simulink library "ox_lib"  (Simulink 7.5)
settings: Solver=ode45  SolverMode=SingleTasking  StartTime=0.0  StopTime=10.0  RelTol=1e-3
PostLoadFcn:
  | % Stub definitions for mask variables
  | delay_depth=16;
  | n_bits=8;
  | bin_pt=7;
libraries: xbsIndex_r4 x493, casper_library x127, casper_library_misc x2, xps_library x2, casper_library_delays x1
(part 1 of 5)
settings Model: Creator=mwagner  LastModifiedBy=jack

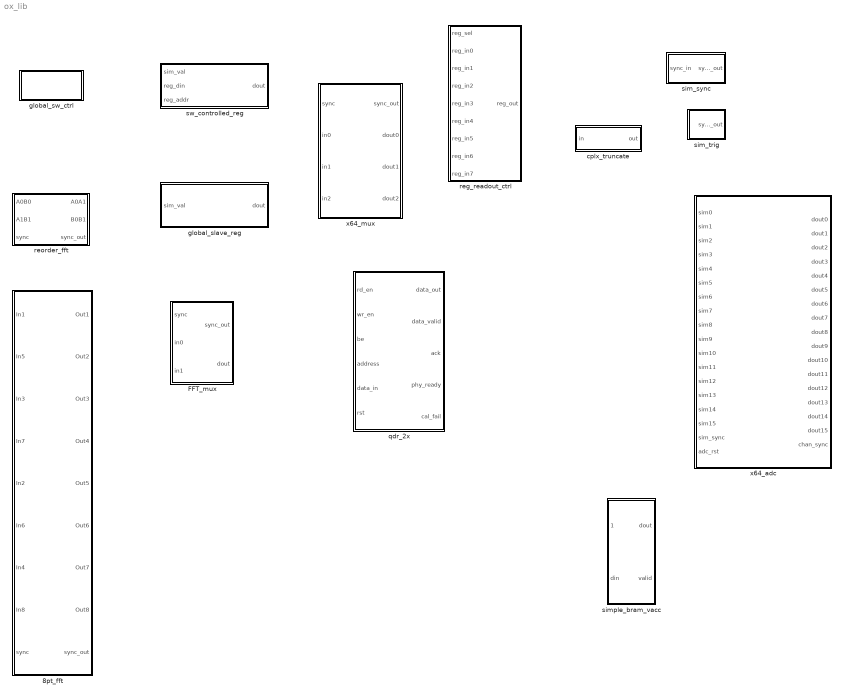
== system ox_lib ==
  8pt_fft : Subsystem
      mask Type: 8pt_fft
      mask Description:
      | Input 8 values and get 8 fourier components!
      | 
      | Simples!
      | 
      | [Latency 24]
  FFT_mux : Subsystem  mask{fft_len=9, fft_inputs=2, bit_width=18, bram_lat=2}
      mask prompts: fft_len "FFT length (2^?)"; fft_inputs "Number of FFT inputs (2^?) -- doesn't yet work for values other than 2"; bit_width "Bit width of samples"; bram_lat "bram latency"
  cplx_truncate : Subsystem  mask{in_bits=19, out_bits=16}
      mask prompts: in_bits "Input bitwidth"; out_bits "Output bitwidth"
  global_slave_reg : Subsystem  mask{reg_name=My Register, data_width=32, latency=0, auto=off, enable_bit=0}
      mask prompts: reg_name "Register Name"; data_width "Data width (bits): 1-32"; latency "Pipelined delay (0 for none)"; auto "Use automatic addressing? (not yet implemented)"; enable_bit "Address Number: 0-31"
      mask init:
      | pipeline_init([gcb '/pipeline1'], 'latency', latency);
      | pipeline_init([gcb '/pipeline2'], 'latency', latency);
      | 
      | fmtstr = sprintf('Name: %s, Number :%d, Latency:%d', reg_name, enable_bit, latency);
      | 
      | set_param(gcb, 'AttributesFormatString', fmtstr);
      settings: AttributesFormatString=Name: My Register, Number :0, Latency:10
  global_sw_ctrl : Subsystem
      settings: PermitHierarchicalResolution=None
      mask Type: global_sw_reg
      mask Description: The beginnings of a lightweight control system for designs with many software registers.
  qdr_2x : Subsystem  Tag=xps:qdr_2x  mask(qdr_2x){which_qdr=qdr0, qdr_awidth=12, use_sniffer=off}
      mask prompts: which_qdr "QDR Chip"; qdr_awidth "Simulation QDR address width"; use_sniffer "Include CPU Interface"
      mask help: Interface to the QDR II SRAM device on ROACH, with 2x multiplexing
      mask init:
      | qdr_2x_mask(gcb);
      mask StyleString: popup(qdr0|qdr1),edit,checkbox
  reg_readout_ctrl : Subsystem  mask{n_registers=8, mux_latency=2}
      mask prompts: n_registers "Number of register inputs"; mux_latency "mux latency"
      mask init:
      | reg_readout_ctrl_init(gcb, ...
      |     'n_registers', n_registers, ...
      |     'mux_latency', mux_latency);
      settings: AttributesFormatString=|
      | n_inputs=8
      | latency=2
  reorder_fft : Subsystem  mask{N=256}
      mask prompts: N "window size"
  sim_sync : Subsystem  mask{delay=1}
      mask prompts: delay "time of pulse (clocks from simulation start)"
  sim_trig : Subsystem  mask{delay=1}
      mask prompts: delay "time of pulse (clocks from simulation start)"
  simple_bram_vacc : Subsystem  mask(simple_bram_vacc){vec_len=8, arith_type=Signed, n_bits=32, bin_pt=0, acc_len=4}
      mask prompts: vec_len "Vector length:"; arith_type "Output type:"; n_bits "Bit width (output):"; bin_pt "Binary point (output):"; acc_len "Accumulation length?"
      mask help:
      | This simple vector accumulator is based on a shift register. It outputs its accumulated vector as soon as it is calculated.
      |
      | (I.e, it does not require a further new acc pulse, and therefore won't break if there are periods of invalid data)
      mask init:
      | simple_bram_vacc_init(gcb, ...
      |     'vec_len', vec_len, ...
      |     'arith_type', arith_type, ...
      |     'n_bits', n_bits, ...
      |     'bin_pt', bin_pt);
      | 
      | fmtstr = sprintf('Acc len: %d', acc_len);
      | set_param(gcb, 'AttributesFormatString', fmtstr);
      settings: AttributesFormatString=Acc len: 4
      mask StyleString: edit,popup(Signed|Unsigned),edit,edit,edit
  sw_controlled_reg : Subsystem  mask{reg_name=My Register, enable_bit=0, data_width=32}
      mask prompts: reg_name "Register Name"; enable_bit "Address Number: 0-31"; data_width "Data width (bits): 1-32"
      mask init:
      | fmtstr = sprintf('Name: %s\nNumber :%d', reg_name, enable_bit);
      | 
      | set_param(gcb, 'AttributesFormatString', fmtstr);
      settings: AttributesFormatString=|
      | Name: My Register
      | Number :0
  x64_adc : Subsystem  Tag=xps:x64_adc  mask(x64_adc){adc_clk_rate=64, spi=off, ctrl_gpio=GPIO_A}
      mask prompts: adc_clk_rate "ADC clock rate (MHz)"; spi "Include SPI interface?"; ctrl_gpio "GPIO bank to use for control signals?"
      mask help: The ADC block converts analog inputs to digital outputs. Every clock cycle, the inputs are sampled and digitized to 8 bit binary point numbers in the range of [-1, 1) and are then output by the adc.
      mask init:
      | x64_adc_mask(gcb);
      mask Help: eval('xlWeb([getenv(''MLIB_ROOT''), ''\doc\html\sys_adc\sys_adc.html''])')
      mask StyleString: edit,checkbox,popup(GPIO_A|GPIO_B)
  x64_mux : Subsystem  mask{fft_len=2, bram_lat=2}
      mask prompts: fft_len "FFT length (2^?)"; bram_lat "bram latency"

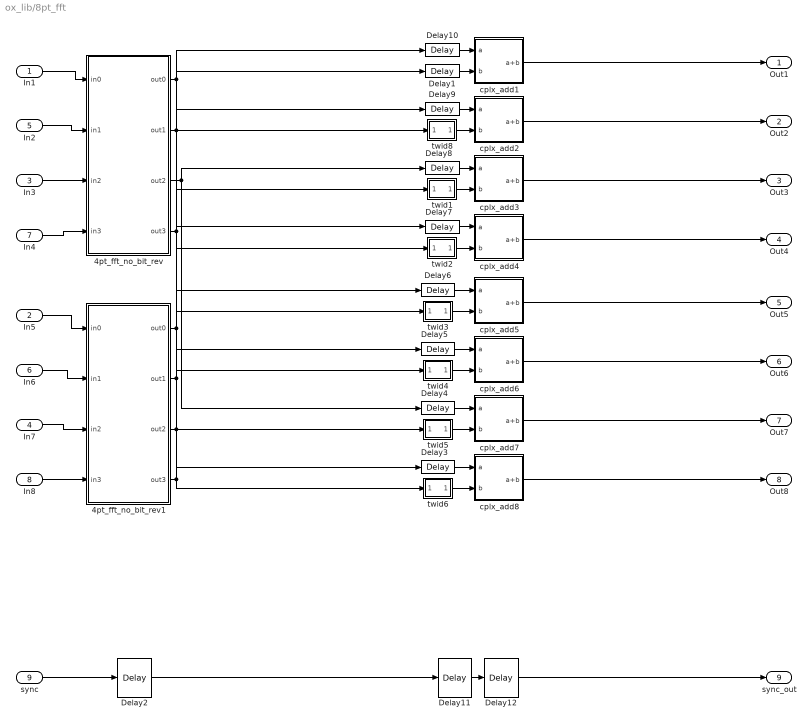
== system ox_lib/8pt_fft ==
  In1 : Inport  OutDataType=sfix(16)  OutScaling=2^0
  In5 : Inport  Port=2  OutDataType=sfix(16)  OutScaling=2^0
  In3 : Inport  Port=3  OutDataType=sfix(16)  OutScaling=2^0
  In7 : Inport  Port=4  OutDataType=sfix(16)  OutScaling=2^0
  In2 : Inport  Port=5  OutDataType=sfix(16)  OutScaling=2^0
  In6 : Inport  Port=6  OutDataType=sfix(16)  OutScaling=2^0
  In4 : Inport  Port=7  OutDataType=sfix(16)  OutScaling=2^0
  In8 : Inport  Port=8  OutDataType=sfix(16)  OutScaling=2^0
  sync : Inport  Port=9  OutDataType=sfix(16)  OutScaling=2^0
  4pt_fft_no_bit_rev : Subsystem
  4pt_fft_no_bit_rev1 : Subsystem
  Delay{1,3..11} (10 alike) : xbsIndex_r4/Delay  en=off  latency=8  dbl_ovrd=off  reg_retiming=off  block_type=delay
      settings: block_version=11.4
  Delay12 : xbsIndex_r4/Delay  en=off  latency=4  dbl_ovrd=off  reg_retiming=off  block_type=delay
      settings: block_version=11.4
  Delay2 : xbsIndex_r4/Delay  en=off  latency=12  dbl_ovrd=off  reg_retiming=off  block_type=delay
      settings: block_version=11.4
  cplx_add1 : Subsystem  AncestorBlock=casper_library/Misc/complex_addsub  mask(cplx_add){BitWidth=8, add_latency=2}
      mask prompts: BitWidth "Bit Wdith"; add_latency "Add Latency"
  cplx_add2 : Subsystem  AncestorBlock=casper_library/Misc/complex_addsub  mask(cplx_add){BitWidth=8, add_latency=2}
      mask prompts: BitWidth "Bit Wdith"; add_latency "Add Latency"
  cplx_add3 : Subsystem  AncestorBlock=casper_library/Misc/complex_addsub  mask(cplx_add){BitWidth=8, add_latency=2}
      mask prompts: BitWidth "Bit Wdith"; add_latency "Add Latency"
  cplx_add4 : Subsystem  AncestorBlock=casper_library/Misc/complex_addsub  mask(cplx_add){BitWidth=8, add_latency=2}
      mask prompts: BitWidth "Bit Wdith"; add_latency "Add Latency"
  cplx_add5 : Subsystem  AncestorBlock=casper_library/Misc/complex_addsub  mask(cplx_add){BitWidth=8, add_latency=2}
      mask prompts: BitWidth "Bit Wdith"; add_latency "Add Latency"
  cplx_add6 : Subsystem  AncestorBlock=casper_library/Misc/complex_addsub  mask(cplx_add){BitWidth=8, add_latency=2}
      mask prompts: BitWidth "Bit Wdith"; add_latency "Add Latency"
  cplx_add7 : Subsystem  AncestorBlock=casper_library/Misc/complex_addsub  mask(cplx_add){BitWidth=8, add_latency=2}
      mask prompts: BitWidth "Bit Wdith"; add_latency "Add Latency"
  cplx_add8 : Subsystem  AncestorBlock=casper_library/Misc/complex_addsub  mask(cplx_add){BitWidth=8, add_latency=2}
      mask prompts: BitWidth "Bit Wdith"; add_latency "Add Latency"
  twid1 : Subsystem  mask{phase=-2*pi/4}
      mask init:
      | fmtstr = sprintf('twiddle_phase: %d', phase);
      | set_param(gcb, 'AttributesFormatString', fmtstr);
      settings: AttributesFormatString=twiddle_phase: -1.570796e+00
  twid2 : Subsystem  mask{phase=-3*pi/4}
      mask init:
      | fmtstr = sprintf('twiddle_phase: %d', phase);
      | set_param(gcb, 'AttributesFormatString', fmtstr);
      settings: AttributesFormatString=twiddle_phase: -2.356194e+00
  twid3 : Subsystem  mask{phase=-4*pi/4}
      mask init:
      | fmtstr = sprintf('twiddle_phase: %d', phase);
      | set_param(gcb, 'AttributesFormatString', fmtstr);
      settings: AttributesFormatString=twiddle_phase: -3.141593e+00
  twid4 : Subsystem  mask{phase=-5*pi/4}
      mask init:
      | fmtstr = sprintf('twiddle_phase: %d', phase);
      | set_param(gcb, 'AttributesFormatString', fmtstr);
      settings: AttributesFormatString=twiddle_phase: -3.926991e+00
  twid5 : Subsystem  mask{phase=-6*pi/4}
      mask init:
      | fmtstr = sprintf('twiddle_phase: %d', phase);
      | set_param(gcb, 'AttributesFormatString', fmtstr);
      settings: AttributesFormatString=twiddle_phase: -4.712389e+00
  twid6 : Subsystem  mask{phase=-7*pi/4}
      mask init:
      | fmtstr = sprintf('twiddle_phase: %d', phase);
      | set_param(gcb, 'AttributesFormatString', fmtstr);
      settings: AttributesFormatString=twiddle_phase: -5.497787e+00
  twid8 : Subsystem  mask{phase=-pi/4}
      mask init:
      | fmtstr = sprintf('twiddle_phase: %d', phase);
      | set_param(gcb, 'AttributesFormatString', fmtstr);
      settings: AttributesFormatString=twiddle_phase: -7.853982e-01
  Out1 : Outport  OutDataType=sfix(16)  OutScaling=2^0
  Out2 : Outport  Port=2  OutDataType=sfix(16)  OutScaling=2^0
  Out3 : Outport  Port=3  OutDataType=sfix(16)  OutScaling=2^0
  Out4 : Outport  Port=4  OutDataType=sfix(16)  OutScaling=2^0
  Out5 : Outport  Port=5  OutDataType=sfix(16)  OutScaling=2^0
  Out6 : Outport  Port=6  OutDataType=sfix(16)  OutScaling=2^0
  Out7 : Outport  Port=7  OutDataType=sfix(16)  OutScaling=2^0
  Out8 : Outport  Port=8  OutDataType=sfix(16)  OutScaling=2^0
  sync_out : Outport  Port=9  OutDataType=sfix(16)  OutScaling=2^0
  wires:
  Delay10/1 -> cplx_add1/1(a)
  Delay9/1 -> cplx_add2/1(a)
  Delay8/1 -> cplx_add3/1(a)
  Delay7/1 -> cplx_add4/1(a)
  Delay6/1 -> cplx_add5/1(a)
  Delay5/1 -> cplx_add6/1(a)
  Delay4/1 -> cplx_add7/1(a)
  Delay3/1 -> cplx_add8/1(a)
  cplx_add8/1(a+b) -> Out8/1
  cplx_add7/1(a+b) -> Out7/1
  cplx_add6/1(a+b) -> Out6/1
  cplx_add5/1(a+b) -> Out5/1
  cplx_add4/1(a+b) -> Out4/1
  cplx_add3/1(a+b) -> Out3/1
  cplx_add2/1(a+b) -> Out2/1
  cplx_add1/1(a+b) -> Out1/1
  twid6/1(Out1) -> cplx_add8/2(b)
  twid5/1(Out1) -> cplx_add7/2(b)
  twid4/1(Out1) -> cplx_add6/2(b)
  twid3/1(Out1) -> cplx_add5/2(b)
  twid2/1(Out1) -> cplx_add4/2(b)
  twid1/1(Out1) -> cplx_add3/2(b)
  twid8/1(Out1) -> cplx_add2/2(b)
  Delay1/1 -> cplx_add1/2(b)
  sync/1 -> Delay2/1
  Delay2/1 -> Delay11/1
  Delay11/1 -> Delay12/1
  Delay12/1 -> sync_out/1
  In1/1 -> 4pt_fft_no_bit_rev/1(in0)
  In5/1 -> 4pt_fft_no_bit_rev1/1(in0)
  In6/1 -> 4pt_fft_no_bit_rev1/2(in1)
  In7/1 -> 4pt_fft_no_bit_rev1/3(in2)
  In8/1 -> 4pt_fft_no_bit_rev1/4(in3)
  4pt_fft_no_bit_rev/1(out0) -> Delay10/1, Delay6/1
  4pt_fft_no_bit_rev/2(out1) -> Delay9/1, Delay5/1
  4pt_fft_no_bit_rev/3(out2) -> Delay8/1, Delay4/1
  4pt_fft_no_bit_rev/4(out3) -> Delay7/1, Delay3/1
  4pt_fft_no_bit_rev1/1(out0) -> twid3/1(In1), Delay1/1
  4pt_fft_no_bit_rev1/2(out1) -> twid4/1(In1), twid8/1(In1)
  4pt_fft_no_bit_rev1/3(out2) -> twid5/1(In1), twid1/1(In1)
  4pt_fft_no_bit_rev1/4(out3) -> twid6/1(In1), twid2/1(In1)
  In2/1 -> 4pt_fft_no_bit_rev/2(in1)
  In3/1 -> 4pt_fft_no_bit_rev/3(in2)
  In4/1 -> 4pt_fft_no_bit_rev/4(in3)

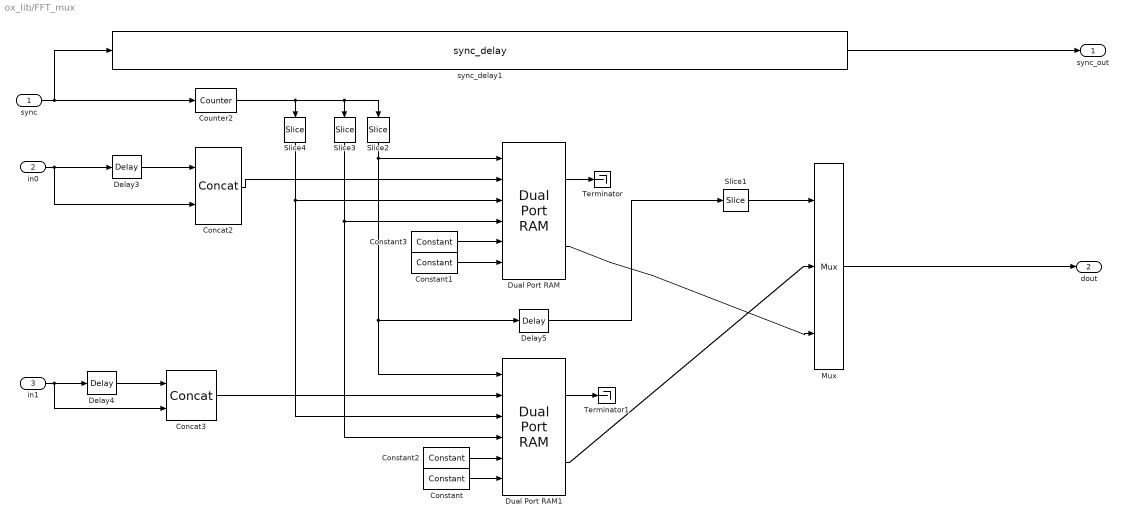
== system ox_lib/FFT_mux ==
  sync : Inport  OutDataType=fixdt(1, 16)  OutScaling=2^0
  in0 : Inport  Port=2  OutDataType=fixdt(1, 16)  OutScaling=2^0
  in1 : Inport  Port=3  OutDataType=fixdt(1, 16)  OutScaling=2^0
  Concat2 : xbsIndex_r4/Concat  num_inputs=2  dbl_ovrd=off  block_type=concat
  Concat3 : xbsIndex_r4/Concat  num_inputs=2  dbl_ovrd=off  block_type=concat
  Constant : xbsIndex_r4/Constant  arith_type=Boolean  const=0  n_bits=16  bin_pt=14  explicit_period=off  period=1  equ=P=C  opselect=C  inp2=PCIN>>17  opr=+  inp1=P  carry=CIN  dbl_ovrd=off  block_type=constant
      settings: block_version=11.4
  Constant1 : xbsIndex_r4/Constant  arith_type=Boolean  const=0  n_bits=16  bin_pt=14  explicit_period=off  period=1  equ=P=C  opselect=C  inp2=PCIN>>17  opr=+  inp1=P  carry=CIN  dbl_ovrd=off  block_type=constant
      settings: block_version=11.4
  Constant2 : xbsIndex_r4/Constant  arith_type=Unsigned  const=0  n_bits=(2^fft_inputs)*bit_width  bin_pt=0  explicit_period=on  period=1  equ=P=C  opselect=C  inp2=PCIN>>17  opr=+  inp1=P  carry=CIN  dbl_ovrd=off  block_type=constant
      settings: block_version=11.4
  Constant3 : xbsIndex_r4/Constant  arith_type=Unsigned  const=0  n_bits=(2^fft_inputs)*bit_width  bin_pt=0  explicit_period=on  period=1  equ=P=C  opselect=C  inp2=PCIN>>17  opr=+  inp1=P  carry=CIN  dbl_ovrd=off  block_type=constant
      settings: block_version=11.4
  Counter2 : xbsIndex_r4/Counter  cnt_type=Free Running  cnt_to=Inf  operation=Up  start_count=0  cnt_by_val=1  arith_type=Unsigned  n_bits=fft_len-fft_inputs+1  bin_pt=0  load_pin=off  rst=on  en=off  explicit_period=on  period=1  dbl_ovrd=off  use_behavioral_HDL=off  implementation=Fabric  block_type=counter
      settings: block_version=11.4
  Delay3 : xbsIndex_r4/Delay  en=off  latency=1  dbl_ovrd=off  reg_retiming=off  block_type=delay
      settings: block_version=11.4
  Delay4 : xbsIndex_r4/Delay  en=off  latency=1  dbl_ovrd=off  reg_retiming=off  block_type=delay
      settings: block_version=11.4
  Delay5 : xbsIndex_r4/Delay  en=off  latency=bram_lat  dbl_ovrd=off  reg_retiming=off  block_type=delay
      settings: block_version=11.4
  Dual Port RAM : xbsIndex_r4/Dual Port RAM  depth=2^(fft_len-fft_inputs)  initVector=0  distributed_mem=Block RAM  init_a=0  init_b=0  rst_a=off  rst_b=off  en_a=off  en_b=off  latency=bram_lat  write_mode_A=Read Before Write  write_mode_B=Read Before Write  dbl_ovrd=off  optimize=Area  use_rpm=on  block_type=dpram
      settings: block_version=11.4
  Dual Port RAM1 : xbsIndex_r4/Dual Port RAM  depth=2^(fft_len-fft_inputs)  initVector=0  distributed_mem=Block RAM  init_a=0  init_b=0  rst_a=off  rst_b=off  en_a=off  en_b=off  latency=bram_lat  write_mode_A=Read Before Write  write_mode_B=Read Before Write  dbl_ovrd=off  optimize=Area  use_rpm=on  block_type=dpram
      settings: block_version=11.4
  Mux : xbsIndex_r4/Mux  inputs=2  en=off  latency=1  precision=Full  arith_type=Unsigned  n_bits=16  bin_pt=14  quantization=Truncate  overflow=Wrap  dbl_ovrd=off  block_type=mux
      settings: block_version=11.4
  Slice1 : xbsIndex_r4/Slice  nbits=1  boolean_output=off  mode=Upper Bit Location + Width  bit1=0  base1=MSB of Input  bit0=0  base0=LSB of Input  dbl_ovrd=off  block_type=slice
  Slice2 : xbsIndex_r4/Slice  nbits=fft_len-fft_inputs  boolean_output=off  mode=Upper Bit Location + Width  bit1=0  base1=MSB of Input  bit0=0  base0=LSB of Input  dbl_ovrd=off  block_type=slice
  Slice3 : xbsIndex_r4/Slice  nbits=fft_len-fft_inputs  boolean_output=off  mode=Lower Bit Location + Width  bit1=0  base1=MSB of Input  bit0=0  base0=LSB of Input  dbl_ovrd=off  block_type=slice
  Slice4 : xbsIndex_r4/Slice  nbits=1  boolean_output=on  mode=Lower Bit Location + Width  bit1=0  base1=MSB of Input  bit0=0  base0=LSB of Input  dbl_ovrd=off  block_type=slice
  Terminator : Terminator
  Terminator1 : Terminator
  sync_delay1 : casper_library/Delays/sync_delay  SystemSampleTime=-1  DelayLen=2^(fft_len-fft_inputs)+bram_lat+1
  sync_out : Outport
  dout : Outport  Port=2
  wires:
  Dual Port RAM1/1 -> Terminator1/1
  Dual Port RAM/1 -> Terminator/1
  Delay5/1 -> Slice1/1
  sync_delay1/1 -> sync_out/1
  Mux/1 -> dout/1
  Slice1/1 -> Mux/1
  Constant3/1 -> Dual Port RAM/5
  Constant2/1 -> Dual Port RAM1/5
  Constant1/1 -> Dual Port RAM/6
  Constant/1 -> Dual Port RAM1/6
  Slice4/1 -> Dual Port RAM1/3, Dual Port RAM/3
  Slice3/1 -> Dual Port RAM1/4, Dual Port RAM/4
  Slice2/1 -> Delay5/1, Dual Port RAM1/1, Dual Port RAM/1
  Counter2/1 -> Slice4/1, Slice3/1, Slice2/1
  sync/1 -> sync_delay1/1, Counter2/1
  Concat3/1 -> Dual Port RAM1/2
  in1/1 -> Delay4/1, Concat3/2
  Delay4/1 -> Concat3/1
  Concat2/1 -> Dual Port RAM/2
  in0/1 -> Delay3/1, Concat2/2
  Delay3/1 -> Concat2/1
  Dual Port RAM/2 -> Mux/3
  Dual Port RAM1/2 -> Mux/2

== system ox_lib/cplx_truncate ==
  in : Inport  OutDataType=sfix(16)  OutScaling=2^0
  c_to_ri : casper_library_misc/c_to_ri  SystemSampleTime=-1  n_bits=in_bits  bin_pt=in_bits-1
      settings: AttributesFormatString=19_18 r/i
  convert_im : xbsIndex_r4/Convert  arith_type="Signed  (2's comp)"  n_bits=out_bits  bin_pt=out_bits-1  quantization=Truncate  overflow=Wrap  latency=0  dbl_ovrd=off  pipeline=on  block_type=convert
      settings: xl_area=[0, 0, 0, 0, 0, 0, 0]  block_version=10.1.3
  convert_re : xbsIndex_r4/Convert  arith_type="Signed  (2's comp)"  n_bits=out_bits  bin_pt=out_bits-1  quantization=Truncate  overflow=Wrap  latency=0  dbl_ovrd=off  pipeline=on  block_type=convert
      settings: xl_area=[0, 0, 0, 0, 0, 0, 0]  block_version=10.1.3
  ri_to_c : casper_library_misc/ri_to_c  SystemSampleTime=-1
  out : Outport  OutDataType=sfix(16)  OutScaling=2^0
  wires:
  convert_im/1 -> ri_to_c/2
  c_to_ri/2 -> convert_im/1
  in/1 -> c_to_ri/1
  ri_to_c/1 -> out/1
  convert_re/1 -> ri_to_c/1
  c_to_ri/1 -> convert_re/1

== system ox_lib/global_slave_reg ==
  sim_val : Inport
  Register : xbsIndex_r4/Register  init=0  rst=off  en=on  dbl_ovrd=off  block_type=register
      settings: block_version=11.4
  Simulation Multiplexer : xbsIndex_r4/Simulation Multiplexer  sim_sel=1  hw_sel=2  block_type=simmux
      settings: infoedit="Distinguish input subsystems as \"simulation only\" and \"generation only\".  The input specified For Simulation will be used during Simulink simulation.  The input specified For Generation will be used during code generation.  This block will typically be used on the output of a HW Co-Simulation, Black Box, or ModelSim subsystem.<br><br>Hardware Notes: This block costs nothing."  block_version=11.4
  data_width : xbsIndex_r4/Slice  nbits=data_width  boolean_output=off  mode=Lower Bit Location + Width  bit1=0  base1=MSB of Input  bit0=0  base0=LSB of Input  dbl_ovrd=off  block_type=slice
  data_width1 : xbsIndex_r4/Slice  nbits=data_width  boolean_output=off  mode=Lower Bit Location + Width  bit1=0  base1=MSB of Input  bit0=0  base0=LSB of Input  dbl_ovrd=off  block_type=slice
  en_sel : xbsIndex_r4/Slice  nbits=1  boolean_output=on  mode=Lower Bit Location + Width  bit1=0  base1=MSB of Input  bit0=enable_bit  base0=LSB of Input  dbl_ovrd=off  block_type=slice
  pipeline1 : casper_library_delays/pipeline  SystemSampleTime=-1  latency=latency
  pipeline2 : casper_library/Delays/pipeline  SystemSampleTime=-1  latency=latency
  simulation_val : xbsIndex_r4/Gateway In  arith_type="Signed  (2's comp)"  n_bits=16  bin_pt=14  quantization="Round  (unbiased: +/- Inf)"  overflow=Saturate  period=1  dbl_ovrd=off  timing_constraint=None  locs_specified=off  LOCs={}  hdl_port=on  block_type=gatewayin
      settings: infoedit="Gateway in block.  Converts inputs of type Simulink integer, double and fixed point to  Xilinx fixed point type.<br><br>Hardware notes:  In hardware these blocks become top level input ports."  block_version=11.4
  dout : Outport
  wires:
  data_width1/1 -> Simulation Multiplexer/1
  Simulation Multiplexer/1 -> dout/1
  sim_val/1 -> simulation_val/1
  data_width/1 -> Register/1
  en_sel/1 -> Register/2
  Register/1 -> Simulation Multiplexer/2
  simulation_val/1 -> data_width1/1
  [reg_addr] -> pipeline2/1
  [reg_data] -> pipeline1/1
  pipeline2/1 -> en_sel/1
  pipeline1/1 -> data_width/1

== system ox_lib/global_sw_ctrl ==
  err_clear_sim10 : Constant  Value=0  OutDataType=sfix(16)  OutScaling=2^0
  err_clear_sim5 : Constant  Value=0  OutDataType=sfix(16)  OutScaling=2^0
  reg_addr : xps_library/software register  Tag=xps:sw_reg  SystemSampleTime=-1  io_dir=From Processor  arith_type=Unsigned  bitwidth=32  bin_pt=0  sample_period=1  gw_name=ox_lib_global_sw_ctrl_reg_addr_user_data_out
      link override b_2x_8a_r310b_base_ant0_user_data_out: arith_type=Unsigned  n_bits=32  bin_pt=0  period=1
      link override r_2x_8a_r310b_base_ant0_user_data_out: arith_type=Unsigned  n_bits=32  bin_pt=0  period=1
      link override r_2x_8a_r311a_base_ant0_user_data_out: arith_type=Unsigned  n_bits=32  bin_pt=0  period=1
      link override r_2x_8a_r311b_1_base_ant0_user_data_out: arith_type=Unsigned  n_bits=32  bin_pt=0  period=1
      link override r_2x_8a_r311b_base_ant0_user_data_out: arith_type=Unsigned  n_bits=32  bin_pt=0  period=1
      link override r_2x_8a_r320a_1_base_ant0_user_data_out: arith_type=Unsigned  n_bits=32  bin_pt=0  period=1
      link override r_2x_8a_r320b_1_base_ant0_user_data_out: arith_type=Unsigned  n_bits=32  bin_pt=0  period=1
      link override r_2x_8a_r320b_base_ant0_user_data_out: arith_type=Unsigned  n_bits=32  bin_pt=0  period=1
      link override r_4f_1x_16a_r322h_base_ant0_user_data_out: arith_type=Unsigned  n_bits=32  bin_pt=0  period=1
      link override r_4f_1x_16a_r322i_base_ant0_user_data_out: arith_type=Unsigned  n_bits=32  bin_pt=0  period=1
      link override r_4f_1x_16a_r322j_base_ant0_user_data_out: arith_type=Unsigned  n_bits=32  bin_pt=0  period=1
      link override r_4f_1x_16a_r322k_base_ant0_user_data_out: arith_type=Unsigned  n_bits=32  bin_pt=0  period=1
      link override r_4f_1x_16a_r322l_base_ant0_user_data_out: arith_type=Unsigned  n_bits=32  bin_pt=0  period=1
      link override r_4f_1x_16a_r322m_base_ant0_user_data_out: arith_type=Unsigned  n_bits=32  bin_pt=0  period=1
      link override r_4f_2x_16a_r320b_base_ant0_user_data_out: arith_type=Unsigned  n_bits=32  bin_pt=0  period=1
      link override r_4f_2x_16a_r321a_base_ant0_user_data_out: arith_type=Unsigned  n_bits=32  bin_pt=0  period=1
      link override r_4f_2x_16a_r322a_base_ant0_user_data_out: arith_type=Unsigned  n_bits=32  bin_pt=0  period=1
      link override r_4f_2x_16a_r322b_base_ant0_user_data_out: arith_type=Unsigned  n_bits=32  bin_pt=0  period=1
      link override r_4f_2x_16a_r322c_base_ant0_user_data_out: arith_type=Unsigned  n_bits=32  bin_pt=0  period=1
      link override r_4f_2x_16a_r322d_base_ant0_user_data_out: arith_type=Unsigned  n_bits=32  bin_pt=0  period=1
      link override r_4f_2x_16a_r322e_base_ant0_user_data_out: arith_type=Unsigned  n_bits=32  bin_pt=0  period=1
      link override r_4f_2x_16a_r322f_base_ant0_user_data_out: arith_type=Unsigned  n_bits=32  bin_pt=0  period=1
      link override r_4f_2x_16a_r322g_base_ant0_user_data_out: arith_type=Unsigned  n_bits=32  bin_pt=0  period=1
      link override r_4f_2x_16a_r322h_base_ant0_user_data_out: arith_type=Unsigned  n_bits=32  bin_pt=0  period=1
      link override r_4f_2x_16a_r322m_base_ant0_user_data_out: arith_type=Unsigned  n_bits=32  bin_pt=0  period=1
      link override r_4f_2x_16a_r323a_base_ant0_user_data_out: arith_type=Unsigned  n_bits=32  bin_pt=0  period=1
      link override r_r311b_xaui_test_base_ant0_user_data_out: arith_type=Unsigned  n_bits=32  bin_pt=0  period=1
  reg_data : xps_library/software register  Tag=xps:sw_reg  SystemSampleTime=-1  io_dir=From Processor  arith_type=Unsigned  bitwidth=32  bin_pt=0  sample_period=1  gw_name=ox_lib_global_sw_ctrl_reg_data_user_data_out
      link override b_2x_8a_r310b_base_ant0_user_data_out: arith_type=Unsigned  n_bits=32  bin_pt=0  period=1
      link override r_2x_8a_r310b_base_ant0_user_data_out: arith_type=Unsigned  n_bits=32  bin_pt=0  period=1
      link override r_2x_8a_r311a_base_ant0_user_data_out: arith_type=Unsigned  n_bits=32  bin_pt=0  period=1
      link override r_2x_8a_r311b_1_base_ant0_user_data_out: arith_type=Unsigned  n_bits=32  bin_pt=0  period=1
      link override r_2x_8a_r311b_base_ant0_user_data_out: arith_type=Unsigned  n_bits=32  bin_pt=0  period=1
      link override r_2x_8a_r320a_1_base_ant0_user_data_out: arith_type=Unsigned  n_bits=32  bin_pt=0  period=1
      link override r_2x_8a_r320b_1_base_ant0_user_data_out: arith_type=Unsigned  n_bits=32  bin_pt=0  period=1
      link override r_2x_8a_r320b_base_ant0_user_data_out: arith_type=Unsigned  n_bits=32  bin_pt=0  period=1
      link override r_4f_1x_16a_r322h_base_ant0_user_data_out: arith_type=Unsigned  n_bits=32  bin_pt=0  period=1
      link override r_4f_1x_16a_r322i_base_ant0_user_data_out: arith_type=Unsigned  n_bits=32  bin_pt=0  period=1
      link override r_4f_1x_16a_r322j_base_ant0_user_data_out: arith_type=Unsigned  n_bits=32  bin_pt=0  period=1
      link override r_4f_1x_16a_r322k_base_ant0_user_data_out: arith_type=Unsigned  n_bits=32  bin_pt=0  period=1
      link override r_4f_1x_16a_r322l_base_ant0_user_data_out: arith_type=Unsigned  n_bits=32  bin_pt=0  period=1
      link override r_4f_1x_16a_r322m_base_ant0_user_data_out: arith_type=Unsigned  n_bits=32  bin_pt=0  period=1
      link override r_4f_2x_16a_r320b_base_ant0_user_data_out: arith_type=Unsigned  n_bits=32  bin_pt=0  period=1
      link override r_4f_2x_16a_r321a_base_ant0_user_data_out: arith_type=Unsigned  n_bits=32  bin_pt=0  period=1
      link override r_4f_2x_16a_r322a_base_ant0_user_data_out: arith_type=Unsigned  n_bits=32  bin_pt=0  period=1
      link override r_4f_2x_16a_r322b_base_ant0_user_data_out: arith_type=Unsigned  n_bits=32  bin_pt=0  period=1
      link override r_4f_2x_16a_r322c_base_ant0_user_data_out: arith_type=Unsigned  n_bits=32  bin_pt=0  period=1
      link override r_4f_2x_16a_r322d_base_ant0_user_data_out: arith_type=Unsigned  n_bits=32  bin_pt=0  period=1
      link override r_4f_2x_16a_r322e_base_ant0_user_data_out: arith_type=Unsigned  n_bits=32  bin_pt=0  period=1
      link override r_4f_2x_16a_r322f_base_ant0_user_data_out: arith_type=Unsigned  n_bits=32  bin_pt=0  period=1
      link override r_4f_2x_16a_r322g_base_ant0_user_data_out: arith_type=Unsigned  n_bits=32  bin_pt=0  period=1
      link override r_4f_2x_16a_r322h_base_ant0_user_data_out: arith_type=Unsigned  n_bits=32  bin_pt=0  period=1
      link override r_4f_2x_16a_r322m_base_ant0_user_data_out: arith_type=Unsigned  n_bits=32  bin_pt=0  period=1
      link override r_4f_2x_16a_r323a_base_ant0_user_data_out: arith_type=Unsigned  n_bits=32  bin_pt=0  period=1
      link override r_r311b_xaui_test_base_ant0_user_data_out: arith_type=Unsigned  n_bits=32  bin_pt=0  period=1
  tag scope: reg_addr=global, reg_data=global
  wires:
  err_clear_sim5/1 -> reg_addr/1
  reg_addr/1 -> [reg_addr]
  err_clear_sim10/1 -> reg_data/1
  reg_data/1 -> [reg_data]
